simulink model "simple_summator"  (Simulink 8.0)
settings: Solver=ode45  StartTime=0.0  StopTime=10.0  RelTol=1e-3
undefined symbols (not defined in the file): DiscIntNeverNeededParam
settings Model: Creator=rstarr  LastModifiedBy=rstarr

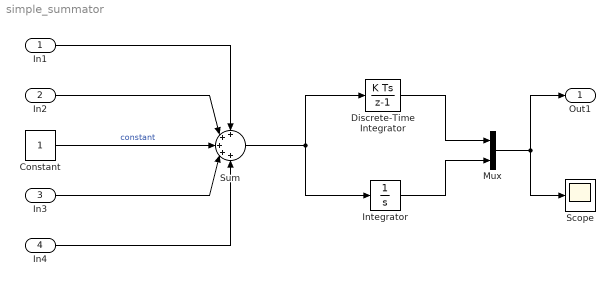
== system simple_summator ==
  In1 : Inport
  In2 : Inport  Port=2
  In3 : Inport  Port=3
  In4 : Inport  Port=4
  Constant : Constant
  Discrete-Time Integrator : DiscreteIntegrator  SampleTime=0.1  ICPrevOutput=DiscIntNeverNeededParam  ICPrevScaledInput=DiscIntNeverNeededParam
  Integrator : Integrator
  Mux : Mux  Inputs=2
  Scope : Scope
  Sum : Sum  Inputs=+++++
  Out1 : Outport
  wires:
  Constant/1 -> Sum/3  "constant"
  In2/1 -> Sum/2
  In3/1 -> Sum/4
  In1/1 -> Sum/1
  In4/1 -> Sum/5
  Sum/1 -> Discrete-Time Integrator/1, Integrator/1
  Integrator/1 -> Mux/2
  Discrete-Time Integrator/1 -> Mux/1
  Mux/1 -> Out1/1, Scope/1
